simulink model "Position_State_Feedback_Simulation"  (R2021b)
settings: Solver=VariableStepAuto  StartTime=0.0  StopTime=15  RelTol=1e-3
libraries: cstblocks x1
settings Model: Creator=UTENTE  LastModifiedBy=UTENTE

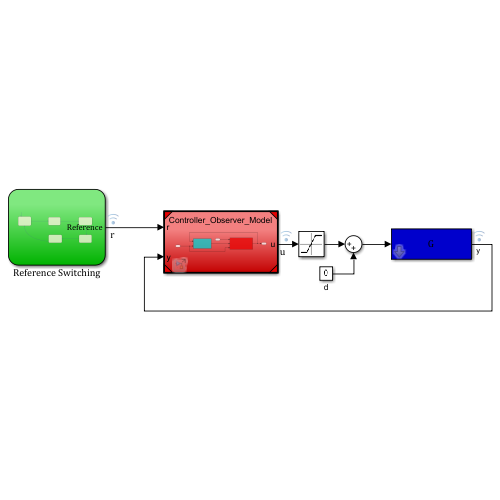
[thumbnail: Simulink's stored preview of the top-level diagram]
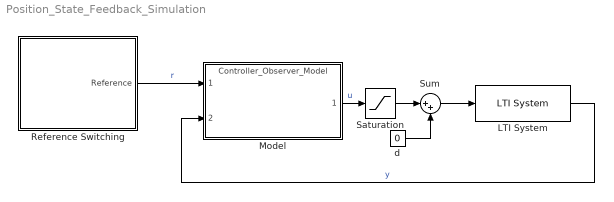
== system Position_State_Feedback_Simulation ==
  LTI System : cstblocks/LTI System  sys=G  IC=[]
  Model : ModelReference  ModelNameDialog=Controller_Observer_Model.slx  SimulationMode=Normal  ModelReferenceVersion=1.47
  Reference Switching : Stateflow chart  TreatAsAtomicUnit=on
  Saturation : Saturate  UpperLimit=12  LowerLimit=-12
  Sum : Sum  Inputs=|++
  d : Constant  Value=0
  wires:
  Model/1 -> Saturation/1  "u"
  Reference Switching/1(Reference) -> Model/1  "r"
  Sum/1 -> LTI System/1
  d/1 -> Sum/2
  LTI System/1 -> Model/2  "y"
  Saturation/1 -> Sum/1

== stateflow chart Position_State_Feedback_Simulation/Reference Switching ==
  state S1
    Reference=0;
  state S2
    Reference=-pi;
  state S3
    Reference=pi;
  state s6
    Reference=0;
  state s5
    Reference=2*pi;
  (default) -> S1
  S1 -> S2 : after(2,sec)
  S2 -> S3 : after(2,sec)
  S3 -> s5 : after(2,sec)
  s6 -> S1 : after(2,sec)
  s5 -> s6 : after(2,sec)
  data: Reference output
